simulink model "myproject_task"  (Simulink 3.00)
undefined symbols (not defined in the file): Double, F64
libraries: mathlib x3, speclib x1, arclib x1

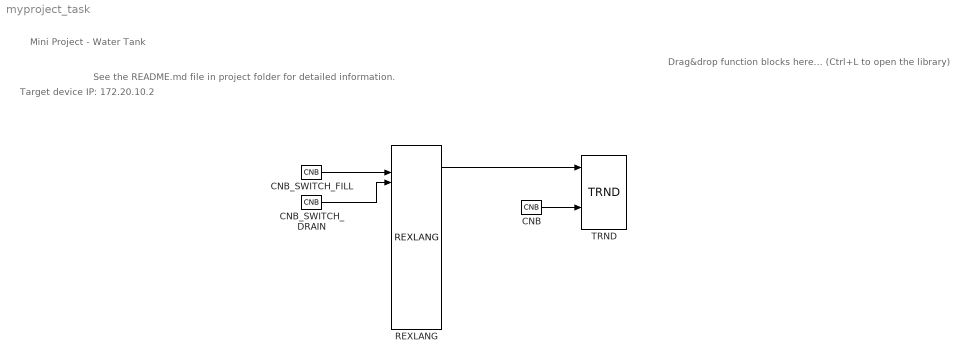
== system myproject_task ==
  note: Drag&drop function blocks here...
      |
      | (Ctrl+L to open the library)
  note: See the README.md file in project folder for detailed information.
  note: Mini Project - Water Tank
  note: Target device IP: 172.20.10.2
  CNB : mathlib/CNB  YCN=on
  CNB_SWITCH_DRAIN : mathlib/CNB  YCN=off
  CNB_SWITCH_FILL : mathlib/CNB  YCN=on
  REXLANG : speclib/REXLANG  srcname=srcfile.st  srctype=2: STL  debug=3: Full check  stack=0  strs=0
  TRND : arclib/TRND  n=4  l=1000  btype=8: Double (F64)  ptype1=1: Store  ptype2=1: Store  ptype3=1: Store  ptype4=1: Store  pfac=1  afac=0  arc=0  id=0  Title=Trend Title  timesrc=1: CORETIMER
  wires:
  CNB/1 -> TRND/5
  CNB_SWITCH_DRAIN/1 -> REXLANG/4
  CNB_SWITCH_FILL/1 -> REXLANG/3
  REXLANG/2 -> TRND/1
